simulink model "Prelab3_Motor_control_with_unity_feedback"  (R2014a)
settings: Solver=ode45  StartTime=0.0  StopTime=10.0  RelTol=1e-3
values from neighbouring files (symbols this model uses):
  K = 19.4    [Lab3code.m]
  K_r = 0    [Lab3code.m]
  T_d = 1    [Lab3code.m]
undefined symbols (not defined in the file or in its folder): B, J, w_r
settings Model: Creator=Matthew  LastModifiedBy=Matthew

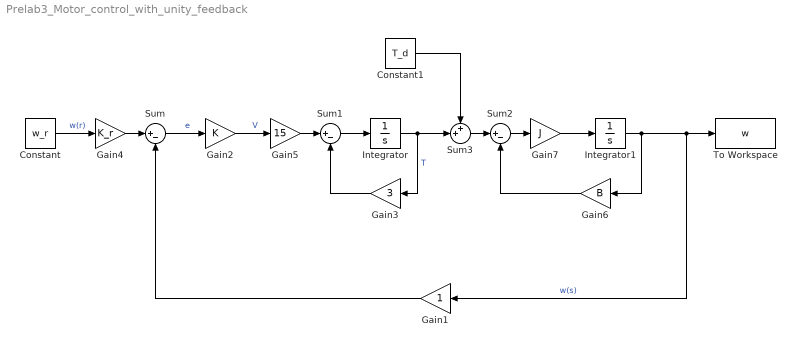
== system Prelab3_Motor_control_with_unity_feedback ==
  Constant : Constant  Value=w_r
  Constant1 : Constant  Value=T_d
  Gain1 : Gain
  Gain2 : Gain  Gain=K
  Gain3 : Gain  Gain=3
  Gain4 : Gain  Gain=K_r
  Gain5 : Gain  Gain=15
  Gain6 : Gain  Gain=B
  Gain7 : Gain  Gain=J
  Integrator : Integrator
  Integrator1 : Integrator
  Sum : Sum  Inputs=|+-
  Sum1 : Sum  Inputs=|+-
  Sum2 : Sum  Inputs=|+-
  Sum3 : Sum  Inputs=++|
  To Workspace : ToWorkspace  VariableName=w  SampleTime=-1
  wires:
  Constant/1 -> Gain4/1  "w(r)"
  Gain4/1 -> Sum/1
  Gain1/1 -> Sum/2
  Sum/1 -> Gain2/1  "e"
  Integrator/1 -> Gain3/1, Sum3/2  "T"
  Gain3/1 -> Sum1/2
  Gain5/1 -> Sum1/1
  Sum1/1 -> Integrator/1
  Gain2/1 -> Gain5/1  "V"
  Sum2/1 -> Gain7/1
  Gain7/1 -> Integrator1/1
  Integrator1/1 -> Gain6/1, Gain1/1, To Workspace/1  "w(s)"
  Sum3/1 -> Sum2/1
  Gain6/1 -> Sum2/2
  Constant1/1 -> Sum3/1
